simulink model "integration_2-1"  (R2023b)
settings: Solver=FixedStepAuto  StartTime=0.0  StopTime=inf  FixedStep=0.01  RelTol=1e-3  EnableMultiTasking=on
InitFcn:
  | params
  | pin_params
undefined symbols (not defined in the file): b, default1, den_Gd, encoder_scale, f, J, Kb, KD, Kf, KI, Km, KP, l, L, num_Gd, r, R, steering, Vlim
libraries: arduinolib x18, arduinosensorlib x8, simulink x2
settings Model: SimulationMode=external  ExtModeTrigDuration=2  Creator=권주성  LastModifiedBy=tkdle
settings SolverCC: AutoInsertRateTranBlk=on
settings OptimizationCC: EnhancedBackFolding=on  PassReuseOutputArgsAs=Individual arguments  ZeroExternalMemoryAtStartup=off  ZeroInternalMemoryAtStartup=off  MaxStackSize=64  OptimizeBlockOrder=speed  DifferentSizesBufferReuse=on  OptimizationCustomize=off  EfficientTunableParamExpr=on
settings DebuggingCC: ParameterPrecisionLossMsg=none  ParameterTunabilityLossMsg=error
settings HardwareCC: ProdBitPerInt=16  ProdBitPerPointer=16  ProdBitPerSizeT=16  ProdBitPerPtrDiffT=16  ProdLargestAtomicFloat=None  ProdWordSize=8  ProdHWDeviceType=Atmel->AVR
settings SFSimCC: MATLABDynamicMemAlloc=off
settings RTWCC: Description=Embedded Coder  SystemTargetFile=ert.tlc  HardwareBoard=Arduino Mega 2560  TemplateMakefile=ert_default_tmf  Toolchain=Arduino AVR  BuildConfiguration=Faster Runs
settings CodeAppCC: ForceParamTrailComments=on  IgnoreCustomStorageClasses=off  OperatorAnnotations=on  SimulinkDataObjDesc=on  SFDataObjDesc=on  InsertBlockDesc=on
settings ERTTargetCC: SupportContinuousTime=on  SupportVariableSizeSignals=on  ExtMode=on  ExtModeTransport=3  ExtModeStaticAlloc=on  ExtModeAutomaticAllocSize=off  ExtModeStaticAllocSize=2048  ExtModeMexFile=ext_xcp  ExtModeMexArgs=0 12 921600  ExtModeIntrfLevel=Level2 - Open

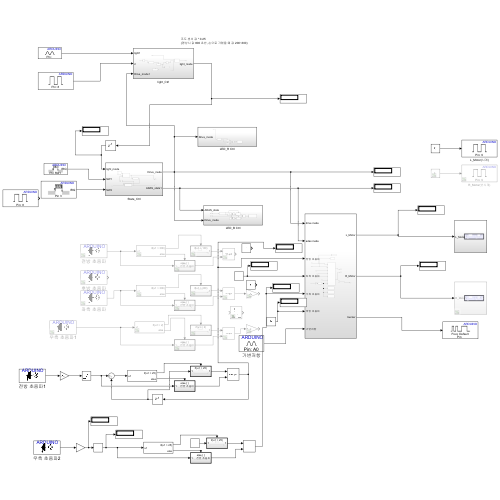
[thumbnail: Simulink's stored preview of the top-level diagram]
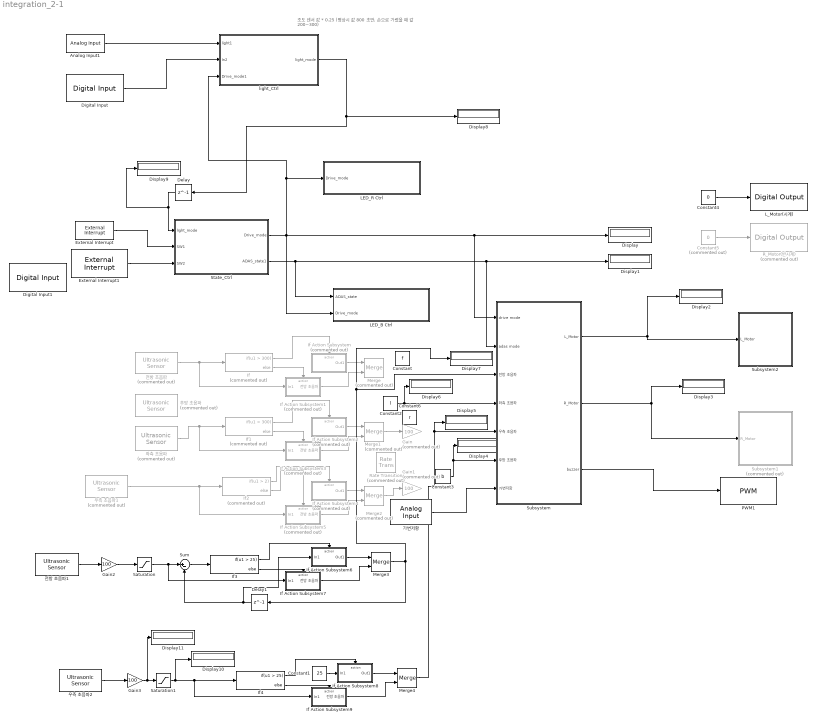
== system integration_2-1 ==
  note: 조도 센서 값 * 0.25
      | (평상시 값 800 초반, 손으로 가렸을 때 값 200~300)
  Analog Input1 : arduinolib/Analog Input  pinNumber=BS  ReadResultsOnly=off  ConversionTriggerSource=Software  ExternalTriggerType=uint32( 0 )  OutputDataType=uint16  EnableConversionCompleteNotify=off  EnableOuputStatus=off  SampleTime=-1  blockPlatform=arduino
  Constant : Constant  Value=f
  Constant1 : Constant  Value=25
  Constant2 : Constant  Value=l
  Constant3 : Constant  Value=b
  Constant4 : Constant  Value=0
  Constant5 : Constant  Commented=on  Value=0
  Constant6 : Constant  Value=r
  Delay : Delay  DelayLength=1
  Delay1 : Delay  DelayLength=1
  Digital Input : arduinolib/Digital Input  pinNumber=SW3  mode=Default  Direction=input  SampleTime=0.1  blockPlatform=arduino
  Digital Input1 : arduinolib/Digital Input  pinNumber=SW2  mode=Default  Direction=input  SampleTime=0.1  blockPlatform=arduino
  Display{,1..11} (12 alike) : Display
  External Interrupt : arduinolib/External Interrupt  Pin=SW1  PullUp=off  Mode=RISING  InterruptSimulationInput=off
  External Interrupt1 : arduinolib/External Interrupt  Pin=3  PullUp=off  Mode=RISING  InterruptSimulationInput=off
  Gain : Gain  Commented=on  Gain=100
  Gain1 : Gain  Commented=on  Gain=100
  Gain2 : Gain  Gain=100
  Gain3 : Gain  Gain=100
  If : If  Commented=on  IfExpression=u1 > 300
  If Action Subsystem : Subsystem  Commented=on  TreatAsAtomicUnit=on
  If Action Subsystem1 : Subsystem  Commented=on  TreatAsAtomicUnit=on
  If Action Subsystem2 : Subsystem  Commented=on  TreatAsAtomicUnit=on
  If Action Subsystem3 : Subsystem  Commented=on  TreatAsAtomicUnit=on
  If Action Subsystem4 : Subsystem  Commented=on  TreatAsAtomicUnit=on
  If Action Subsystem5 : Subsystem  Commented=on  TreatAsAtomicUnit=on
  If Action Subsystem6 : Subsystem  TreatAsAtomicUnit=on
  If Action Subsystem7 : Subsystem  TreatAsAtomicUnit=on
  If Action Subsystem8 : Subsystem  TreatAsAtomicUnit=on
  If Action Subsystem9 : Subsystem  TreatAsAtomicUnit=on
  If1 : If  Commented=on  IfExpression=u1 > 300
  If2 : If  Commented=on  IfExpression=u1 > 2
  If3 : If  IfExpression=u1 > 25
  If4 : If  IfExpression=u1 > 25
  LED_B Ctrl : Subsystem
  LED_R Ctrl : Subsystem
  L_Motor(시계) : arduinolib/Digital Output  pinNumber=Motor_L_Direction  Direction=output  blockPlatform=arduino
  Merge : Merge  Commented=on
  Merge1 : Merge  Commented=on
  Merge2 : Merge  Commented=on
  Merge3 : Merge
  Merge4 : Merge
  PWM1 : arduinolib/PWM  pinNumber=Buzzer  frequencyType=Default  desiredFrequency=490.2  achievableFrequency=490.2
  R_Motor(반시계) : arduinolib/Digital Output  Commented=on  pinNumber=Motor_R_Direction  Direction=output  blockPlatform=arduino
  Rate Transition : RateTransition  Commented=on  Integrity=off  OutPortSampleTime=0.01
  Saturation : Saturate  UpperLimit=30  LowerLimit=0
  Saturation1 : Saturate  UpperLimit=30
  State_Ctrl : Subsystem
  Subsystem : Subsystem
  Subsystem1 : Subsystem  Commented=on
  Subsystem2 : Subsystem
  Sum : Sum  Inputs=|+-
  light_Ctrl : Subsystem
  가변저항 : arduinolib/Analog Input  pinNumber=0  ReadResultsOnly=off  ConversionTriggerSource=Software  ExternalTriggerType=uint32( 0 )  OutputDataType=uint16  EnableConversionCompleteNotify=off  EnableOuputStatus=off  SampleTime=-1  blockPlatform=arduino
  우측 초음파1 : arduinosensorlib/Ultrasonic Sensor  Commented=on  NumSignalPins=2  TrigPin=R_Triger  EchoPin=R_Echo  SignalPin=3  SampleTime_=0.01  blockPlatform=ARDUINO
  우측 초음파2 : arduinosensorlib/Ultrasonic Sensor  NumSignalPins=2  TrigPin=R_Triger  EchoPin=R_Echo  SignalPin=3  SampleTime_=0.01  blockPlatform=ARDUINO
  전방 초음파 : arduinosensorlib/Ultrasonic Sensor  Commented=on  NumSignalPins=2  TrigPin=F_Triger  EchoPin=F_Echo  SignalPin=3  SampleTime_=0.01  blockPlatform=ARDUINO
  전방 초음파1 : arduinosensorlib/Ultrasonic Sensor  NumSignalPins=2  TrigPin=F_Triger  EchoPin=F_Echo  SignalPin=3  SampleTime_=0.01  blockPlatform=ARDUINO
  좌측 초음파 : arduinosensorlib/Ultrasonic Sensor  Commented=on  NumSignalPins=2  TrigPin=L_Triger  EchoPin=L_Echo  SignalPin=3  SampleTime_=0.01  blockPlatform=ARDUINO
  후방 초음파 : arduinosensorlib/Ultrasonic Sensor  Commented=on  NumSignalPins=2  TrigPin=B_Triger  EchoPin=B_Echo  SignalPin=3  SampleTime_=0.01  blockPlatform=ARDUINO
  wires:
  light_Ctrl/1(light_mode) -> Display8/1, Delay/1
  Analog Input1/1 -> light_Ctrl/1(light1)
  Delay/1 -> Display9/1, State_Ctrl/1(light_mode)
  State_Ctrl/2(ADAS_state1) -> LED_B Ctrl/1(ADAS_state), Display1/1, Subsystem/2(adas mode)
  External Interrupt/1 -> State_Ctrl/2(SW1)
  State_Ctrl/1(Drive_mode) -> Subsystem/1(drive mode), Display/1, light_Ctrl/3(Drive_mode1), LED_R Ctrl/1(Drive_mode), LED_B Ctrl/2(Drive_mode)
  가변저항/1 -> Subsystem/7(가변저항)
  Subsystem/3(buzzer) -> PWM1/1
  Subsystem/2(R_Motor) -> Subsystem1/1(R_Motor), Display3/1
  Merge1/1 -> Gain/1
  Constant2/1 -> Subsystem/4(좌측 초음파), Display6/1
  Subsystem/1(L_Motor) -> Display2/1, Subsystem2/1(L_Motor)
  External Interrupt1/1 -> State_Ctrl/3(SW2)
  Digital Input/1 -> light_Ctrl/2(In2)
  Constant4/1 -> L_Motor(시계)/1
  Constant5/1 -> R_Motor(반시계)/1
  전방 초음파/1 -> If Action Subsystem1/1(In1), If/1
  If/1 -> If Action Subsystem/Action
  If/2 -> If Action Subsystem1/Action
  If Action Subsystem/1(Out1) -> Merge/1
  If Action Subsystem1/1(전방 초음파) -> Merge/2
  좌측 초음파/1 -> If Action Subsystem3/1(In1), If1/1
  If1/1 -> If Action Subsystem2/Action
  If1/2 -> If Action Subsystem3/Action
  If Action Subsystem2/1(Out1) -> Merge1/1
  If Action Subsystem3/1(전방 초음파) -> Merge1/2
  If Action Subsystem5/1(전방 초음파) -> Merge2/2
  If Action Subsystem4/1(Out1) -> Merge2/1
  If2/2 -> If Action Subsystem5/Action
  If2/1 -> If Action Subsystem4/Action
  Merge2/1 -> Gain1/1
  우측 초음파1/1 -> If Action Subsystem5/1(In1), If2/1
  전방 초음파1/1 -> Gain2/1
  Gain2/1 -> Saturation/1
  Saturation/1 -> If Action Subsystem7/1(In1), Sum/1
  Merge3/1 -> Subsystem/3(전방 초음파), Display7/1, Delay1/1
  Delay1/1 -> If Action Subsystem6/1(In1), Sum/2
  Sum/1 -> If3/1
  If3/1 -> If Action Subsystem6/Action
  If3/2 -> If Action Subsystem7/Action
  If Action Subsystem6/1(Out1) -> Merge3/1
  If Action Subsystem7/1(전방 초음파) -> Merge3/2
  Constant3/1 -> Display4/1, Subsystem/6(후방 초음파)
  우측 초음파2/1 -> Gain3/1
  If Action Subsystem8/1(Out1) -> Merge4/1
  If4/1 -> If Action Subsystem8/Action
  If Action Subsystem9/1(전방 초음파) -> Merge4/2
  Saturation1/1 -> Display10/1, If4/1, If Action Subsystem9/1(In1)
  Gain3/1 -> Display11/1, Saturation1/1
  Merge4/1 -> Display5/1, Subsystem/5(우측 초음파)
  If4/2 -> If Action Subsystem9/Action
  Constant1/1 -> If Action Subsystem8/1(In1)

== system integration_2-1/If Action Subsystem ==
  Action Port : ActionPort  ActionPortLabel=if(u1 > 100)
  Constant : Constant  Value=f
  Out1 : Outport
  wires:
  Constant/1 -> Out1/1

== system integration_2-1/If Action Subsystem1 ==
  In1 : Inport
  Action Port : ActionPort  ActionPortLabel=else
  전방 초음파 : Outport
  wires:
  In1/1 -> 전방 초음파/1

== system integration_2-1/If Action Subsystem2 ==
  Action Port : ActionPort  ActionPortLabel=if(u1 > 300)
  Constant : Constant  Value=300
  Out1 : Outport
  wires:
  Constant/1 -> Out1/1

== system integration_2-1/If Action Subsystem3 ==
  In1 : Inport
  Action Port : ActionPort  ActionPortLabel=else
  전방 초음파 : Outport
  wires:
  In1/1 -> 전방 초음파/1

== system integration_2-1/If Action Subsystem4 ==
  Action Port : ActionPort  ActionPortLabel=if(u1 > 2)
  Constant : Constant  Value=2
  Out1 : Outport
  wires:
  Constant/1 -> Out1/1

== system integration_2-1/If Action Subsystem5 ==
  In1 : Inport
  Action Port : ActionPort  ActionPortLabel=else
  전방 초음파 : Outport
  wires:
  In1/1 -> 전방 초음파/1

== system integration_2-1/If Action Subsystem6 ==
  In1 : Inport
  Action Port : ActionPort  ActionPortLabel=if(u1 > 25)
  Out1 : Outport
  wires:
  In1/1 -> Out1/1

== system integration_2-1/If Action Subsystem7 ==
  In1 : Inport
  Action Port : ActionPort  ActionPortLabel=else
  전방 초음파 : Outport
  wires:
  In1/1 -> 전방 초음파/1

== system integration_2-1/If Action Subsystem8 ==
  In1 : Inport
  Action Port : ActionPort  ActionPortLabel=if(u1 > 25)
  Out1 : Outport
  wires:
  In1/1 -> Out1/1

== system integration_2-1/If Action Subsystem9 ==
  In1 : Inport
  Action Port : ActionPort  ActionPortLabel=else
  전방 초음파 : Outport
  wires:
  In1/1 -> 전방 초음파/1

== system integration_2-1/LED_B Ctrl ==
  ADAS_state : Inport
  Drive_mode : Inport  Port=2
  Constant : Constant
  Digital Output : arduinolib/Digital Output  pinNumber=LED1_B  Direction=output  blockPlatform=arduino
  If Action Subsystem1 : Subsystem  TreatAsAtomicUnit=on
  If Action Subsystem3 : Subsystem  TreatAsAtomicUnit=on
  If1 : If  IfExpression=u1 ==1
  Merge : Merge
  Product : Product
  Product1 : Product
  Pulse Generator : DiscretePulseGenerator  PulseType=Time based  PulseWidth=50
  wires:
  If1/2 -> If Action Subsystem3/Action
  If Action Subsystem1/1(Out1) -> Merge/1
  ADAS_state/1 -> If1/1
  If1/1 -> If Action Subsystem1/Action
  Merge/1 -> Digital Output/1
  If Action Subsystem3/1(Out1) -> Merge/2
  Drive_mode/1 -> Product/1, Product1/2
  Pulse Generator/1 -> Product/2
  Constant/1 -> Product1/1
  Product1/1 -> If Action Subsystem1/1(Input)
  Product/1 -> If Action Subsystem3/1(Input)

== system integration_2-1/LED_R Ctrl ==
  Drive_mode : Inport
  Digital Output : arduinolib/Digital Output  pinNumber=LED1_R  Direction=output  blockPlatform=arduino
  If Action Subsystem1 : Subsystem  TreatAsAtomicUnit=on
  If Action Subsystem3 : Subsystem  TreatAsAtomicUnit=on
  If1 : If  IfExpression=u1 ==1
  Merge : Merge
  wires:
  If1/2 -> If Action Subsystem3/Action
  If Action Subsystem1/1(Out1) -> Merge/1
  Drive_mode/1 -> If1/1
  If1/1 -> If Action Subsystem1/Action
  Merge/1 -> Digital Output/1
  If Action Subsystem3/1(Out1) -> Merge/2

== system integration_2-1/State_Ctrl ==
  light_mode : Inport
  SW1 : Inport  Port=2
  SW2 : Inport  Port=3
  ADAS_state : Subsystem
  Delay : Delay  DelayLength=1
  If : If  IfExpression=u1 ==1  ShowElse=off
  drive_mode : Subsystem
  Drive_mode : Outport
  ADAS_state1 : Outport  Port=2
  wires:
  If/1 -> ADAS_state/1(In1)
  drive_mode/1(D_mode) -> If/1, Drive_mode/1
  ADAS_state/1(ADAS_state) -> Delay/1, ADAS_state1/1
  SW1/1 -> drive_mode/2(sw1)
  Delay/1 -> drive_mode/3(A_state)
  light_mode/1 -> drive_mode/1(light_mode)
  SW2/1 -> ADAS_state/2(In2)

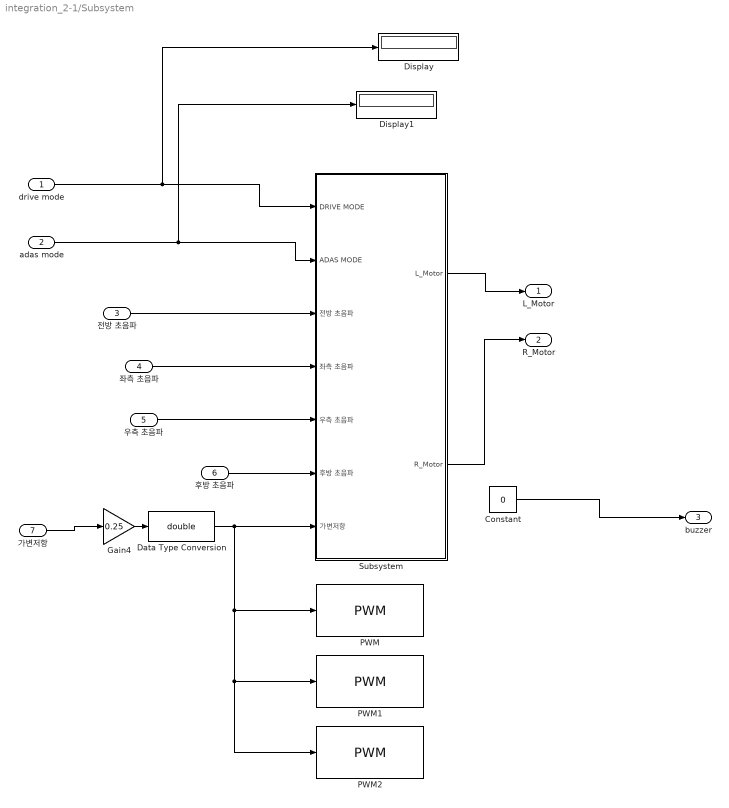
== system integration_2-1/Subsystem ==
  drive mode : Inport
  adas mode : Inport  Port=2
  전방 초음파 : Inport  Port=3
  좌측 초음파 : Inport  Port=4
  우측 초음파 : Inport  Port=5
  후방 초음파 : Inport  Port=6
  가변저항 : Inport  Port=7
  Constant : Constant  Value=0
  Data Type Conversion : DataTypeConversion  OutDataTypeStr=double  SaturateOnIntegerOverflow=off  RndMeth=Floor
  Display : Display
  Display1 : Display
  Gain4 : Gain  Gain=0.25
  PWM : arduinolib/PWM  pinNumber=RGB_LED_1  frequencyType=Default  desiredFrequency=490.2  achievableFrequency=490.2
  PWM1 : arduinolib/PWM  pinNumber=RGB_LED_2  frequencyType=Default  desiredFrequency=490.2  achievableFrequency=490.2
  PWM2 : arduinolib/PWM  pinNumber=RGB_LED_3  frequencyType=Default  desiredFrequency=490.2  achievableFrequency=490.2
  Subsystem : Subsystem
  L_Motor : Outport
  R_Motor : Outport  Port=2
  buzzer : Outport  Port=3
  wires:
  drive mode/1 -> Subsystem/1(DRIVE MODE), Display/1
  adas mode/1 -> Subsystem/2(ADAS MODE), Display1/1
  Constant/1 -> buzzer/1
  가변저항/1 -> Gain4/1
  Gain4/1 -> Data Type Conversion/1
  Data Type Conversion/1 -> Subsystem/7(가변저항), PWM2/1, PWM1/1, PWM/1
  Subsystem/1(L_Motor) -> L_Motor/1
  Subsystem/2(R_Motor) -> R_Motor/1
  전방 초음파/1 -> Subsystem/3(전방 초음파)
  좌측 초음파/1 -> Subsystem/4(좌측 초음파)
  우측 초음파/1 -> Subsystem/5(우측 초음파)
  후방 초음파/1 -> Subsystem/6(후방 초음파)

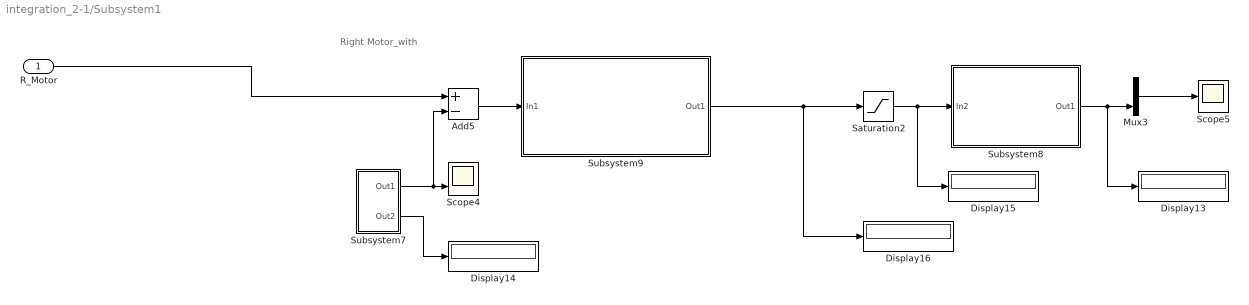
== system integration_2-1/Subsystem1 ==
  note: Right Motor_with
  R_Motor : Inport
  Add5 : Sum  Inputs=+-
  Display{13..16} (4 alike) : Display
  Mux3 : Mux  Inputs=2
  Saturation2 : Saturate  UpperLimit=12  LowerLimit=0
  Scope4 : Scope  NumInputPorts=2
  Scope5 : Scope
  Subsystem7 : Subsystem
  Subsystem8 : Subsystem
  Subsystem9 : Subsystem
  wires:
  Mux3/1 -> Scope5/1
  Saturation2/1 -> Subsystem8/1(In2), Display15/1
  Subsystem9/1(Out1) -> Display16/1, Saturation2/1
  Subsystem8/1(Out1) -> Display13/1, Mux3/2
  Subsystem7/1(Out1) -> Add5/2, Scope4/2
  Subsystem7/2(Out2) -> Display14/1
  Add5/1 -> Subsystem9/1(In1)
  R_Motor/1 -> Add5/1

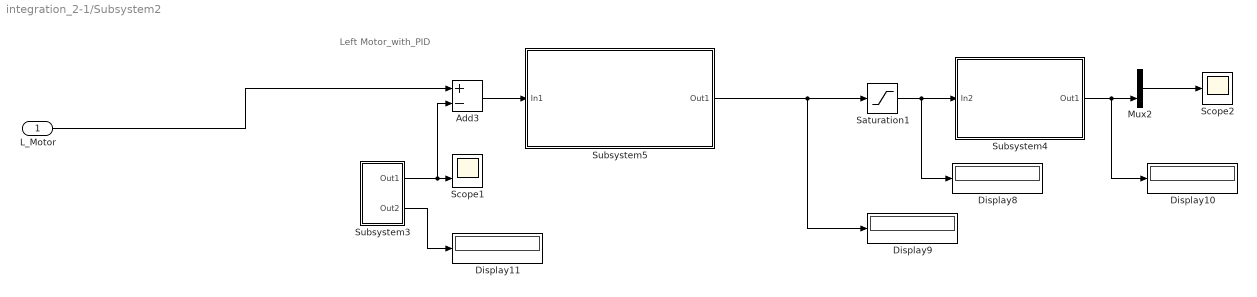
== system integration_2-1/Subsystem2 ==
  note: Left Motor_with_PID
  L_Motor : Inport
  Add3 : Sum  Inputs=+-
  Display{8..11} (4 alike) : Display
  Mux2 : Mux  Inputs=2
  Saturation1 : Saturate  UpperLimit=12  LowerLimit=0
  Scope1 : Scope  NumInputPorts=2
  Scope2 : Scope
  Subsystem3 : Subsystem
  Subsystem4 : Subsystem
  Subsystem5 : Subsystem
  wires:
  Mux2/1 -> Scope2/1
  Saturation1/1 -> Subsystem4/1(In2), Display8/1
  Subsystem5/1(Out1) -> Display9/1, Saturation1/1
  Subsystem3/2(Out2) -> Display11/1
  Add3/1 -> Subsystem5/1(In1)
  Subsystem3/1(Out1) -> Add3/2, Scope1/2
  Subsystem4/1(Out1) -> Display10/1, Mux2/2
  L_Motor/1 -> Add3/1

== system integration_2-1/light_Ctrl ==
  light1 : Inport
  In2 : Inport  Port=2
  Drive_mode1 : Inport  Port=3
  Display1 : Display
  Function-Call Subsystem1 : Subsystem  Commented=on  TreatAsAtomicUnit=on
  If : If  IfExpression=u1 == 0  ShowElse=off
  If Action Subsystem : Subsystem  TreatAsAtomicUnit=on
  Rate Transition : RateTransition  Integrity=off
  Rate Transition1 : RateTransition  Integrity=off  OutPortSampleTime=0.2
  Subsystem : Subsystem
  light_mode : Outport
  wires:
  If Action Subsystem/1(Out1) -> Display1/1, Rate Transition/1
  In2/1 -> Rate Transition1/1
  Rate Transition/1 -> Subsystem/2(sw3)
  Drive_mode1/1 -> Subsystem/3(Drive_mode1)
  light1/1 -> Subsystem/1(light1)
  Subsystem/1(light_mode) -> light_mode/1
  If/1 -> If Action Subsystem/Action
  Rate Transition1/1 -> If/1

== system integration_2-1/LED_B Ctrl/If Action Subsystem1 ==
  Input : Inport
  Action Port : ActionPort  ActionPortLabel=if(u1 ==1)
  Out1 : Outport
  wires:
  Input/1 -> Out1/1

== system integration_2-1/LED_B Ctrl/If Action Subsystem3 ==
  Input : Inport
  Action Port : ActionPort  ActionPortLabel=else
  Out1 : Outport
  wires:
  Input/1 -> Out1/1

== system integration_2-1/LED_R Ctrl/If Action Subsystem1 ==
  Action Port : ActionPort  ActionPortLabel=if(u1 ==1)
  Constant : Constant
  Out1 : Outport
  wires:
  Constant/1 -> Out1/1

== system integration_2-1/LED_R Ctrl/If Action Subsystem3 ==
  Action Port : ActionPort  ActionPortLabel=else
  Constant : Constant  Value=0
  Out1 : Outport
  wires:
  Constant/1 -> Out1/1

== system integration_2-1/State_Ctrl/ADAS_state ==
  In1 : Inport
  In2 : Inport  Port=2
  If Action Subsystem : Subsystem  TreatAsAtomicUnit=on
  Rate Transition2 : RateTransition  Integrity=off
  SW2 : Subsystem
  ADAS_state : Outport
  wires:
  In1/1 -> If Action Subsystem/Action
  If Action Subsystem/1(ADAS_state) -> ADAS_state/1
  In2/1 -> SW2/Trigger
  SW2/1(SW2) -> Rate Transition2/1
  Rate Transition2/1 -> If Action Subsystem/1(sw2)

== system integration_2-1/State_Ctrl/drive_mode ==
  light_mode : Inport
  sw1 : Inport  Port=2
  A_state : Inport  Port=3
  Chart : Stateflow chart  TreatAsAtomicUnit=on
  Rate Transition : RateTransition  Integrity=off
  SW1 : Subsystem
  D_mode : Outport
  wires:
  SW1/1(Output) -> Rate Transition/1
  Rate Transition/1 -> Chart/1(sw1)
  Chart/1(drive_mode) -> D_mode/1
  sw1/1 -> SW1/Trigger
  A_state/1 -> Chart/3(A_state)
  light_mode/1 -> Chart/2(light_mode)

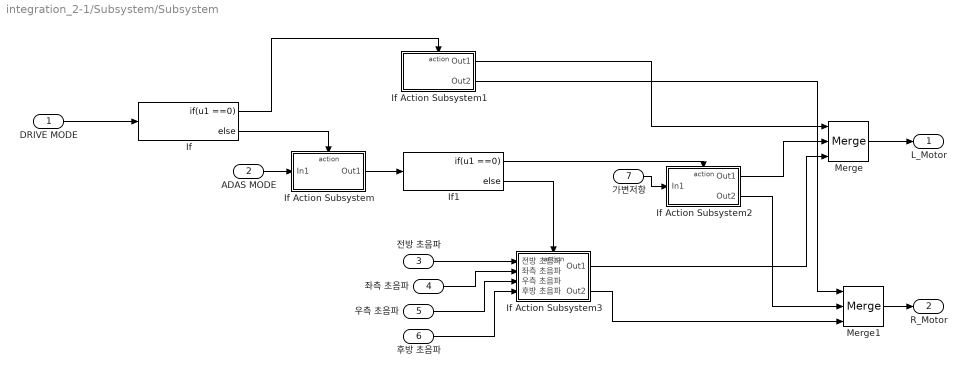
== system integration_2-1/Subsystem/Subsystem ==
  DRIVE MODE : Inport
  ADAS MODE : Inport  Port=2
  전방 초음파 : Inport  Port=3
  좌측 초음파 : Inport  Port=4
  우측 초음파 : Inport  Port=5
  후방 초음파 : Inport  Port=6
  가변저항 : Inport  Port=7
  If : If  IfExpression=u1 ==0
  If Action Subsystem : Subsystem  TreatAsAtomicUnit=on
  If Action Subsystem1 : Subsystem  TreatAsAtomicUnit=on
  If Action Subsystem2 : Subsystem  TreatAsAtomicUnit=on
  If Action Subsystem3 : Subsystem  TreatAsAtomicUnit=on
  If1 : If  IfExpression=u1 ==0
  Merge : Merge  Inputs=3
  Merge1 : Merge  Inputs=3
  L_Motor : Outport
  R_Motor : Outport  Port=2
  wires:
  DRIVE MODE/1 -> If/1
  If/2 -> If Action Subsystem/Action
  If/1 -> If Action Subsystem1/Action
  ADAS MODE/1 -> If Action Subsystem/1(In1)
  If Action Subsystem/1(Out1) -> If1/1
  If1/1 -> If Action Subsystem2/Action
  가변저항/1 -> If Action Subsystem2/1(In1)
  If1/2 -> If Action Subsystem3/Action
  If Action Subsystem1/1(Out1) -> Merge/1
  If Action Subsystem2/1(Out1) -> Merge/2
  If Action Subsystem3/1(Out1) -> Merge/3
  If Action Subsystem1/2(Out2) -> Merge1/1
  If Action Subsystem2/2(Out2) -> Merge1/2
  If Action Subsystem3/2(Out2) -> Merge1/3
  Merge/1 -> L_Motor/1
  Merge1/1 -> R_Motor/1
  전방 초음파/1 -> If Action Subsystem3/1(전방 초음파)
  좌측 초음파/1 -> If Action Subsystem3/2(좌측 초음파)
  우측 초음파/1 -> If Action Subsystem3/3(우측 초음파)
  후방 초음파/1 -> If Action Subsystem3/4(후방 초음파)

== system integration_2-1/Subsystem1/Subsystem7 ==
  Data Type Conversion1 : DataTypeConversion  OutDataTypeStr=int32  SaturateOnIntegerOverflow=off  RndMeth=Floor
  Discrete Transfer Fcn : DiscreteTransferFcn  Numerator=num_Gd  Denominator=den_Gd
  Discrete Derivative : simulink/Discrete/Discrete Derivative  gainval=1.0  ICPrevScaledInput=0.0  OutMin=[]  OutMax=[]  OutDataType=fixdt(1, 16)  OutScaling=2^-10  DoSatur=off
  Display : Display
  Encoder : arduinosensorlib/Encoder  InputA=R_Encoder_A  InputB=R_Encoder_B  Mode=No reset  SampleTime=-1
  Gain1 : Gain  Gain=encoder_scale
  Gain2 : Gain  Gain=60/(2*pi)
  Out1 : Outport
  Out2 : Outport  Port=2
  wires:
  Gain1/1 -> Display/1, Gain2/1, Data Type Conversion1/1
  Encoder/1 -> Discrete Derivative/1
  Gain2/1 -> Out2/1
  Data Type Conversion1/1 -> Discrete Transfer Fcn/1
  Discrete Derivative/1 -> Gain1/1
  Discrete Transfer Fcn/1 -> Out1/1

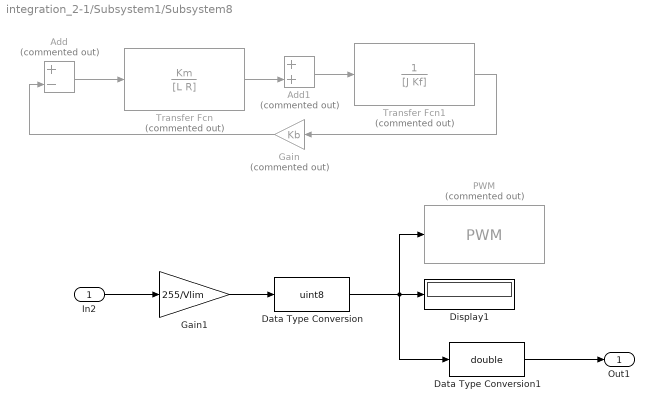
== system integration_2-1/Subsystem1/Subsystem8 ==
  In2 : Inport
  Add : Sum  Commented=on  Inputs=+-
  Add1 : Sum  Commented=on
  Data Type Conversion : DataTypeConversion  OutDataTypeStr=uint8  SaturateOnIntegerOverflow=off  RndMeth=Floor
  Data Type Conversion1 : DataTypeConversion  OutDataTypeStr=double  SaturateOnIntegerOverflow=off  RndMeth=Floor
  Display1 : Display
  Gain : Gain  Commented=on  Gain=Kb
  Gain1 : Gain  Gain=255/Vlim
  PWM : arduinolib/PWM  Commented=on  pinNumber=Motor_R_control  frequencyType=Default  desiredFrequency=490.2  achievableFrequency=490.2
  Transfer Fcn : TransferFcn  Commented=on  Numerator=Km  Denominator=[L R]
  Transfer Fcn1 : TransferFcn  Commented=on  Numerator=1  Denominator=[J Kf]
  Out1 : Outport
  wires:
  ? -> Add/1
  ? -> Add1/1
  Add/1 -> Transfer Fcn/1
  Add1/1 -> Transfer Fcn1/1
  Transfer Fcn/1 -> Add1/2
  Gain/1 -> Add/2
  Transfer Fcn1/1 -> Gain/1
  In2/1 -> Gain1/1
  Gain1/1 -> Data Type Conversion/1
  Data Type Conversion1/1 -> Out1/1
  Data Type Conversion/1 -> Data Type Conversion1/1, Display1/1, PWM/1

== system integration_2-1/Subsystem1/Subsystem9 ==
  In1 : Inport
  Derivative2 : Derivative
  Gain1 : Gain  Gain=KI
  Gain2 : Gain  Gain=KP
  Gain3 : Gain  Gain=KD
  Integrator2 : Integrator
  Subtract2 : Sum  Inputs=+++
  Out1 : Outport
  wires:
  Gain1/1 -> Integrator2/1
  Gain2/1 -> Subtract2/2
  Integrator2/1 -> Subtract2/1
  In1/1 -> Gain2/1, Gain3/1, Gain1/1
  Derivative2/1 -> Subtract2/3
  Gain3/1 -> Derivative2/1
  Subtract2/1 -> Out1/1

== system integration_2-1/Subsystem2/Subsystem3 ==
  Data Type Conversion1 : DataTypeConversion  OutDataTypeStr=int32  SaturateOnIntegerOverflow=off  RndMeth=Floor
  Discrete Transfer Fcn : DiscreteTransferFcn  Numerator=num_Gd  Denominator=den_Gd
  Discrete Derivative : simulink/Discrete/Discrete Derivative  gainval=1.0  ICPrevScaledInput=0.0  OutMin=[]  OutMax=[]  OutDataType=fixdt(1, 16)  OutScaling=2^-10  DoSatur=off
  Display : Display
  Encoder : arduinosensorlib/Encoder  InputA=L_Encoder_A  InputB=L_Encoder_B  Mode=No reset  SampleTime=-1
  Gain1 : Gain  Gain=encoder_scale
  Gain2 : Gain  Gain=60/(2*pi)
  Out1 : Outport
  Out2 : Outport  Port=2
  wires:
  Gain1/1 -> Display/1, Gain2/1, Data Type Conversion1/1
  Encoder/1 -> Discrete Derivative/1
  Gain2/1 -> Out2/1
  Data Type Conversion1/1 -> Discrete Transfer Fcn/1
  Discrete Derivative/1 -> Gain1/1
  Discrete Transfer Fcn/1 -> Out1/1

== system integration_2-1/Subsystem2/Subsystem4 ==
  In2 : Inport
  Add : Sum  Commented=on  Inputs=+-
  Add1 : Sum  Commented=on
  Data Type Conversion : DataTypeConversion  OutDataTypeStr=uint8  SaturateOnIntegerOverflow=off  RndMeth=Floor
  Data Type Conversion1 : DataTypeConversion  OutDataTypeStr=double  SaturateOnIntegerOverflow=off  RndMeth=Floor
  Display1 : Display
  Gain : Gain  Commented=on  Gain=Kb
  Gain1 : Gain  Gain=255/Vlim
  PWM : arduinolib/PWM  pinNumber=Motor_L_Control  frequencyType=Default  desiredFrequency=490.2  achievableFrequency=490.2
  Transfer Fcn : TransferFcn  Commented=on  Numerator=Km  Denominator=[L R]
  Transfer Fcn1 : TransferFcn  Commented=on  Numerator=1  Denominator=[J Kf]
  Out1 : Outport
  wires:
  ? -> Add/1
  ? -> Add1/1
  Add/1 -> Transfer Fcn/1
  Add1/1 -> Transfer Fcn1/1
  Transfer Fcn/1 -> Add1/2
  Gain/1 -> Add/2
  Transfer Fcn1/1 -> Gain/1
  In2/1 -> Gain1/1
  Gain1/1 -> Data Type Conversion/1
  Data Type Conversion1/1 -> Out1/1
  Data Type Conversion/1 -> Data Type Conversion1/1, Display1/1, PWM/1

== system integration_2-1/Subsystem2/Subsystem5 ==
  In1 : Inport
  Derivative2 : Derivative
  Gain1 : Gain  Gain=KI
  Gain2 : Gain  Gain=KP
  Gain3 : Gain  Gain=KD
  Integrator2 : Integrator
  Subtract2 : Sum  Inputs=+++
  Out1 : Outport
  wires:
  Gain1/1 -> Integrator2/1
  Gain2/1 -> Subtract2/2
  Integrator2/1 -> Subtract2/1
  In1/1 -> Gain2/1, Gain3/1, Gain1/1
  Derivative2/1 -> Subtract2/3
  Gain3/1 -> Derivative2/1
  Subtract2/1 -> Out1/1

== system integration_2-1/light_Ctrl/Function-Call Subsystem1 ==
  function : TriggerPort  TriggerType=function-call  VariantControl=(inherit)
  Constant : Constant
  Constant1 : Constant  Value=3
  Delay : Delay  DelayLength=1
  Mod : Math  Operator=mod
  Sum : Sum  Inputs=|++
  Output : Outport
  wires:
  Constant/1 -> Sum/1
  Delay/1 -> Sum/2
  Constant1/1 -> Mod/2
  Sum/1 -> Delay/1, Mod/1
  Mod/1 -> Output/1

== system integration_2-1/light_Ctrl/If Action Subsystem ==
  Action Port : ActionPort  ActionPortLabel=if(u1 == 0)
  Constant : Constant
  Constant1 : Constant  Value=3
  Delay : Delay  DelayLength=1
  Mod : Math  Operator=mod
  Plus : Sum
  Out1 : Outport
  wires:
  Mod/1 -> Out1/1, Delay/1
  Constant/1 -> Plus/1
  Delay/1 -> Plus/2
  Plus/1 -> Mod/1
  Constant1/1 -> Mod/2

== system integration_2-1/light_Ctrl/Subsystem ==
  light1 : Inport
  sw3 : Inport  Port=2
  Drive_mode1 : Inport  Port=3
  Chart1 : Stateflow chart  TreatAsAtomicUnit=on
  Subsystem : Subsystem
  light_mode : Outport
  wires:
  Chart1/1(light_mode) -> Subsystem/2(light_mode), light_mode/1
  light1/1 -> Subsystem/1(light)
  sw3/1 -> Chart1/1(sw3)
  Drive_mode1/1 -> Chart1/2(Drive_mode)

== system integration_2-1/State_Ctrl/ADAS_state/If Action Subsystem ==
  sw2 : Inport
  Action Port : ActionPort  ActionPortLabel=if(u1 ==1)
  Chart : Stateflow chart  TreatAsAtomicUnit=on
  ADAS_state : Outport
  wires:
  sw2/1 -> Chart/1(sw2)
  Chart/1(ADAS_state) -> ADAS_state/1

== system integration_2-1/State_Ctrl/ADAS_state/SW2 ==
  function : TriggerPort  TriggerType=function-call  VariantControl=(inherit)
  Constant : Constant
  Constant1 : Constant  Value=2
  Delay : Delay  DelayLength=1  InitialCondition=0
  Mod : Math  Operator=mod
  Sum : Sum  Inputs=|++
  SW2 : Outport
  wires:
  Sum/1 -> Delay/1, Mod/1
  Constant1/1 -> Mod/2
  Mod/1 -> SW2/1
  Constant/1 -> Sum/1
  Delay/1 -> Sum/2

== system integration_2-1/State_Ctrl/drive_mode/SW1 ==
  function : TriggerPort  TriggerType=function-call  VariantControl=(inherit)
  Constant : Constant
  Constant1 : Constant  Value=2
  Delay : Delay  DelayLength=1
  Mod : Math  Operator=mod
  Sum : Sum  Inputs=|++
  Output : Outport
  wires:
  Constant/1 -> Sum/1
  Sum/1 -> Delay/1, Mod/1
  Constant1/1 -> Mod/2
  Delay/1 -> Sum/2
  Mod/1 -> Output/1

== system integration_2-1/Subsystem/Subsystem/If Action Subsystem ==
  In1 : Inport
  Action Port : ActionPort  ActionPortLabel=else
  Out1 : Outport
  wires:
  In1/1 -> Out1/1

== system integration_2-1/Subsystem/Subsystem/If Action Subsystem1 ==
  Action Port : ActionPort  ActionPortLabel=if(u1 ==0)
  Constant : Constant  Value=0
  Constant1 : Constant  Value=0
  Out1 : Outport
  Out2 : Outport  Port=2
  wires:
  Constant/1 -> Out1/1
  Constant1/1 -> Out2/1

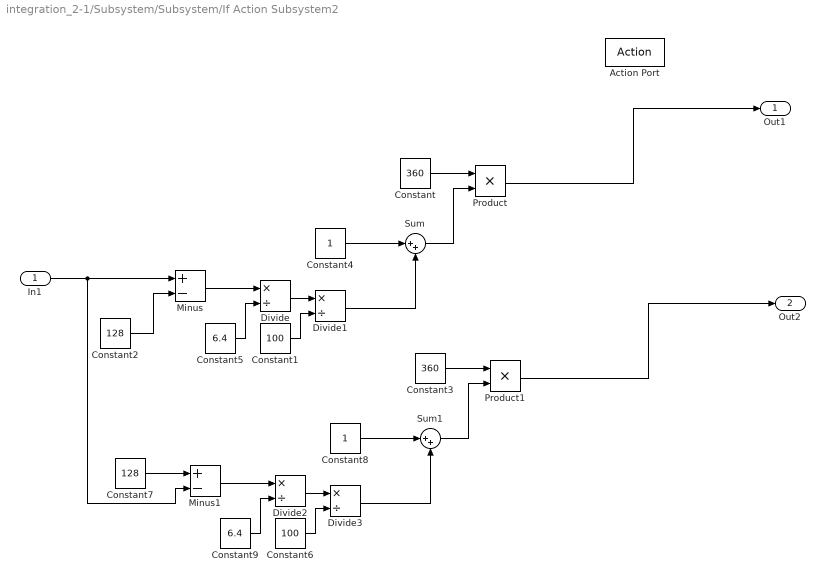
== system integration_2-1/Subsystem/Subsystem/If Action Subsystem2 ==
  In1 : Inport
  Action Port : ActionPort  ActionPortLabel=if(u1 ==0)
  Constant : Constant  Value=360
  Constant1 : Constant  Value=100
  Constant2 : Constant  Value=128
  Constant3 : Constant  Value=360
  Constant4 : Constant
  Constant5 : Constant  Value=6.4
  Constant6 : Constant  Value=100
  Constant7 : Constant  Value=128
  Constant8 : Constant
  Constant9 : Constant  Value=6.4
  Divide{,1..3} (4 alike) : Product  Inputs=*/
  Minus : Sum  Inputs=+-
  Minus1 : Sum  Inputs=+-
  Product : Product
  Product1 : Product
  Sum : Sum  Inputs=|++
  Sum1 : Sum  Inputs=|++
  Out1 : Outport
  Out2 : Outport  Port=2
  wires:
  Product/1 -> Out1/1
  Constant/1 -> Product/1
  In1/1 -> Minus/1, Minus1/2
  Constant2/1 -> Minus/2
  Minus/1 -> Divide/1
  Constant5/1 -> Divide/2
  Divide/1 -> Divide1/1
  Constant1/1 -> Divide1/2
  Constant4/1 -> Sum/1
  Divide1/1 -> Sum/2
  Sum/1 -> Product/2
  Constant7/1 -> Minus1/1
  Minus1/1 -> Divide2/1
  Constant3/1 -> Product1/1
  Constant9/1 -> Divide2/2
  Divide2/1 -> Divide3/1
  Divide3/1 -> Sum1/2
  Product1/1 -> Out2/1
  Constant6/1 -> Divide3/2
  Sum1/1 -> Product1/2
  Constant8/1 -> Sum1/1

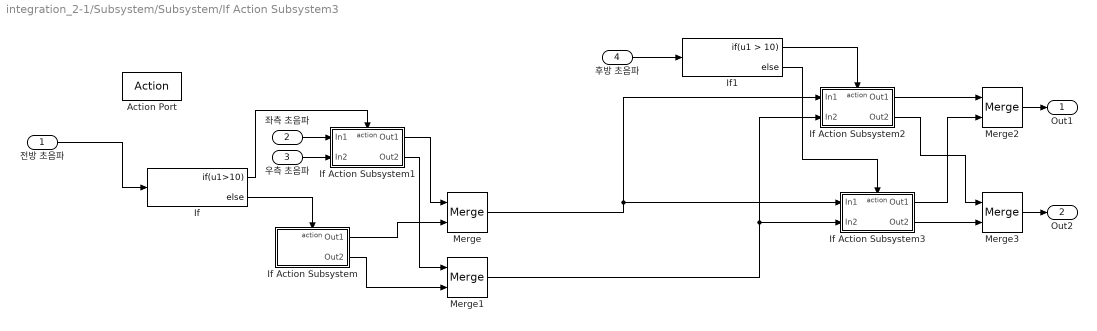
== system integration_2-1/Subsystem/Subsystem/If Action Subsystem3 ==
  전방 초음파 : Inport
  좌측 초음파 : Inport  Port=2
  우측 초음파 : Inport  Port=3
  후방 초음파 : Inport  Port=4
  Action Port : ActionPort  ActionPortLabel=else
  If : If  IfExpression=u1>10
  If Action Subsystem : Subsystem  TreatAsAtomicUnit=on
  If Action Subsystem1 : Subsystem  TreatAsAtomicUnit=on
  If Action Subsystem2 : Subsystem  TreatAsAtomicUnit=on
  If Action Subsystem3 : Subsystem  TreatAsAtomicUnit=on
  If1 : If  IfExpression=u1 > 10
  Merge{,1..3} (4 alike) : Merge
  Out1 : Outport
  Out2 : Outport  Port=2
  wires:
  If/2 -> If Action Subsystem/Action
  전방 초음파/1 -> If/1
  If/1 -> If Action Subsystem1/Action
  If Action Subsystem1/1(Out1) -> Merge/1
  If Action Subsystem/1(Out1) -> Merge/2
  Merge/1 -> If Action Subsystem3/1(In1), If Action Subsystem2/1(In1)
  If Action Subsystem1/2(Out2) -> Merge1/1
  If Action Subsystem/2(Out2) -> Merge1/2
  Merge1/1 -> If Action Subsystem3/2(In2), If Action Subsystem2/2(In2)
  좌측 초음파/1 -> If Action Subsystem1/1(In1)
  우측 초음파/1 -> If Action Subsystem1/2(In2)
  후방 초음파/1 -> If1/1
  If1/1 -> If Action Subsystem2/Action
  If1/2 -> If Action Subsystem3/Action
  If Action Subsystem2/1(Out1) -> Merge2/1
  If Action Subsystem3/1(Out1) -> Merge2/2
  If Action Subsystem3/2(Out2) -> Merge3/2
  If Action Subsystem2/2(Out2) -> Merge3/1
  Merge2/1 -> Out1/1
  Merge3/1 -> Out2/1

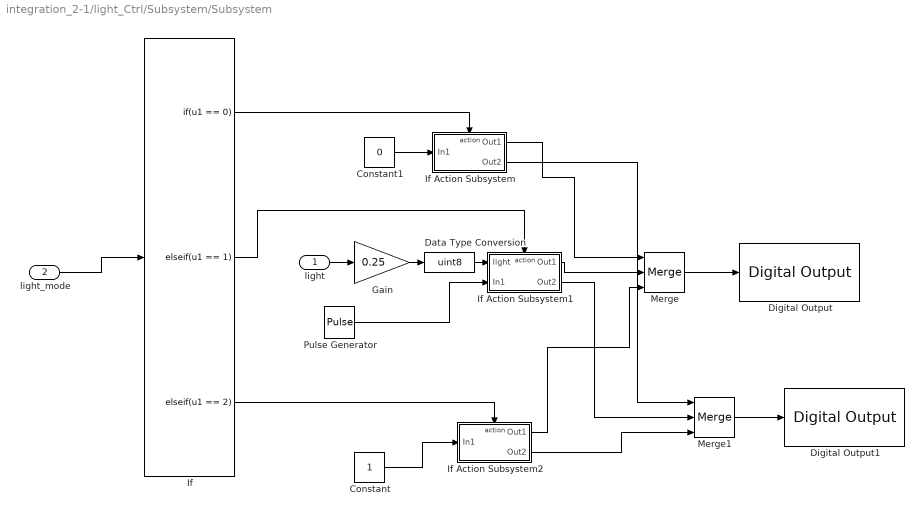
== system integration_2-1/light_Ctrl/Subsystem/Subsystem ==
  light : Inport
  light_mode : Inport  Port=2
  Constant : Constant
  Constant1 : Constant  Value=0
  Data Type Conversion : DataTypeConversion  OutDataTypeStr=uint8  SaturateOnIntegerOverflow=off  RndMeth=Floor
  Digital Output : arduinolib/Digital Output  pinNumber=LED2_R  Direction=output  blockPlatform=arduino
  Digital Output1 : arduinolib/Digital Output  pinNumber=LED2_B  Direction=output  blockPlatform=arduino
  Gain : Gain  Gain=0.25
  If : If  IfExpression=u1 == 0  ElseIfExpressions=u1 == 1, u1 == 2  ShowElse=off
  If Action Subsystem : Subsystem  TreatAsAtomicUnit=on
  If Action Subsystem1 : Subsystem  TreatAsAtomicUnit=on
  If Action Subsystem2 : Subsystem  TreatAsAtomicUnit=on
  Merge : Merge  Inputs=3
  Merge1 : Merge  Inputs=3
  Pulse Generator : DiscretePulseGenerator  PulseType=Time based  Period=0.2  PulseWidth=50
  wires:
  light_mode/1 -> If/1
  If/1 -> If Action Subsystem/Action
  If/2 -> If Action Subsystem1/Action
  If/3 -> If Action Subsystem2/Action
  Constant1/1 -> If Action Subsystem/1(In1)
  Constant/1 -> If Action Subsystem2/1(In1)
  If Action Subsystem/1(Out1) -> Merge/1
  If Action Subsystem1/1(Out1) -> Merge/2
  If Action Subsystem2/1(Out1) -> Merge/3
  Merge/1 -> Digital Output/1
  light/1 -> Gain/1
  Gain/1 -> Data Type Conversion/1
  Data Type Conversion/1 -> If Action Subsystem1/1(light)
  Pulse Generator/1 -> If Action Subsystem1/2(In1)
  If Action Subsystem1/2(Out2) -> Merge1/2
  If Action Subsystem/2(Out2) -> Merge1/1
  If Action Subsystem2/2(Out2) -> Merge1/3
  Merge1/1 -> Digital Output1/1

== system integration_2-1/Subsystem/Subsystem/If Action Subsystem3/If Action Subsystem ==
  Action Port : ActionPort  ActionPortLabel=else
  Constant : Constant  Value=0
  Constant1 : Constant  Value=0
  Out1 : Outport
  Out2 : Outport  Port=2
  wires:
  Constant1/1 -> Out2/1
  Constant/1 -> Out1/1

== system integration_2-1/Subsystem/Subsystem/If Action Subsystem3/If Action Subsystem1 ==
  In1 : Inport
  In2 : Inport  Port=2
  Action Port : ActionPort  ActionPortLabel=if(u1>10)
  If : If  NumInputs=2  IfExpression=(u1<10)&(u2<10)  ElseIfExpressions=u1<10,u2<10
  If Action Subsystem : Subsystem  TreatAsAtomicUnit=on
  If Action Subsystem1 : Subsystem  TreatAsAtomicUnit=on
  If Action Subsystem2 : Subsystem  TreatAsAtomicUnit=on
  If Action Subsystem3 : Subsystem  TreatAsAtomicUnit=on
  Merge : Merge  Inputs=4
  Merge1 : Merge  Inputs=4
  Out1 : Outport
  Out2 : Outport  Port=2
  wires:
  In1/1 -> If Action Subsystem1/1(In3), If Action Subsystem/1(In3), If/1
  If/1 -> If Action Subsystem/Action
  In2/1 -> If Action Subsystem2/1(In3), If Action Subsystem/2(In4), If/2
  If/2 -> If Action Subsystem1/Action
  If/3 -> If Action Subsystem2/Action
  If/4 -> If Action Subsystem3/Action
  If Action Subsystem/1(Out1) -> Merge/1
  If Action Subsystem1/1(Out2) -> Merge/2
  If Action Subsystem2/1(Out2) -> Merge/3
  If Action Subsystem3/1(Out1) -> Merge/4
  If Action Subsystem/2(Out2) -> Merge1/1
  If Action Subsystem1/2(Out3) -> Merge1/2
  If Action Subsystem2/2(Out3) -> Merge1/3
  If Action Subsystem3/2(Out2) -> Merge1/4
  Merge/1 -> Out1/1
  Merge1/1 -> Out2/1

== system integration_2-1/Subsystem/Subsystem/If Action Subsystem3/If Action Subsystem2 ==
  In1 : Inport
  In2 : Inport  Port=2
  Action Port : ActionPort  ActionPortLabel=if(u1 > 10)
  Out1 : Outport
  Out2 : Outport  Port=2
  wires:
  In1/1 -> Out1/1
  In2/1 -> Out2/1

== system integration_2-1/Subsystem/Subsystem/If Action Subsystem3/If Action Subsystem3 ==
  In1 : Inport
  In2 : Inport  Port=2
  Action Port : ActionPort  ActionPortLabel=else
  Gain : Gain  Gain=1.2
  Gain1 : Gain  Gain=1.2
  Out1 : Outport
  Out2 : Outport  Port=2
  wires:
  In1/1 -> Gain/1
  Gain/1 -> Out1/1
  In2/1 -> Gain1/1
  Gain1/1 -> Out2/1

== system integration_2-1/light_Ctrl/Subsystem/Subsystem/If Action Subsystem ==
  In1 : Inport
  Action Port : ActionPort  ActionPortLabel=if(u1 == 0)
  Out1 : Outport
  Out2 : Outport  Port=2
  wires:
  In1/1 -> Out2/1, Out1/1

== system integration_2-1/light_Ctrl/Subsystem/Subsystem/If Action Subsystem1 ==
  light : Inport
  In1 : Inport  Port=2
  Action Port : ActionPort  ActionPortLabel=elseif(u1 == 1)
  Constant : Constant
  Constant1 : Constant  Value=0
  If : If  IfExpression=u1 <= 150
  If Action Subsystem : Subsystem  TreatAsAtomicUnit=on
  If Action Subsystem1 : Subsystem  TreatAsAtomicUnit=on
  Merge : Merge
  Out1 : Outport
  Out2 : Outport  Port=2
  wires:
  light/1 -> If/1
  Constant/1 -> If Action Subsystem/1(In1)
  Constant1/1 -> If Action Subsystem1/1(In1)
  If/1 -> If Action Subsystem/Action
  If/2 -> If Action Subsystem1/Action
  If Action Subsystem/1(Out1) -> Merge/1
  If Action Subsystem1/1(Out1) -> Merge/2
  Merge/1 -> Out1/1
  In1/1 -> Out2/1

== system integration_2-1/light_Ctrl/Subsystem/Subsystem/If Action Subsystem2 ==
  In1 : Inport
  Action Port : ActionPort  ActionPortLabel=elseif( u1 == 2)
  Out1 : Outport
  Out2 : Outport  Port=2
  wires:
  In1/1 -> Out2/1, Out1/1

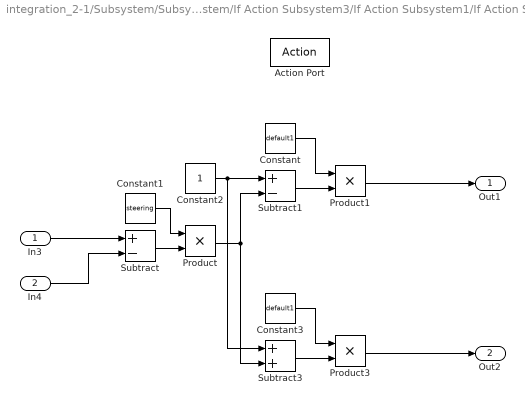
== system integration_2-1/Subsystem/Subsystem/If Action Subsystem3/If Action Subsystem1/If Action Subsystem ==
  In3 : Inport
  In4 : Inport  Port=2
  Action Port : ActionPort  ActionPortLabel=if((u1<10)&(u2<10))
  Constant : Constant  Value=default1
  Constant1 : Constant  Value=steering
  Constant2 : Constant
  Constant3 : Constant  Value=default1
  Product : Product
  Product1 : Product
  Product3 : Product
  Subtract : Sum  Inputs=+-
  Subtract1 : Sum  Inputs=+-
  Subtract3 : Sum
  Out1 : Outport
  Out2 : Outport  Port=2
  wires:
  Subtract/1 -> Product/2
  Constant1/1 -> Product/1
  Subtract1/1 -> Product1/2
  Product/1 -> Subtract1/2, Subtract3/2
  Constant/1 -> Product1/1
  Product1/1 -> Out1/1
  Subtract3/1 -> Product3/2
  Constant2/1 -> Subtract3/1, Subtract1/1
  In4/1 -> Subtract/2
  Constant3/1 -> Product3/1
  In3/1 -> Subtract/1
  Product3/1 -> Out2/1

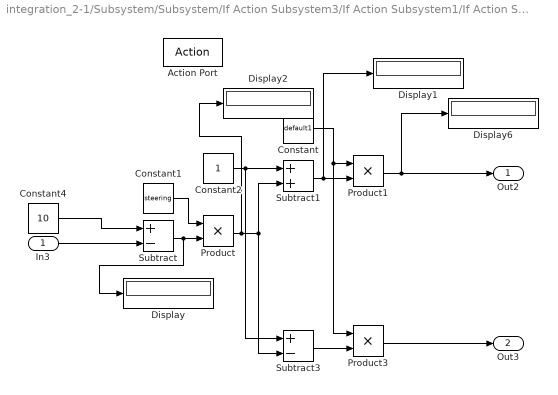
== system integration_2-1/Subsystem/Subsystem/If Action Subsystem3/If Action Subsystem1/If Action Subsystem1 ==
  In3 : Inport
  Action Port : ActionPort  ActionPortLabel=elseif(u1<10)
  Constant : Constant  Value=default1
  Constant1 : Constant  Value=steering
  Constant2 : Constant
  Constant4 : Constant  Value=10
  Display{,1..2,6} (4 alike) : Display
  Product : Product  OutDataTypeStr=double  RndMeth=Convergent
  Product1 : Product  OutDataTypeStr=double  RndMeth=Convergent
  Product3 : Product  OutDataTypeStr=double  RndMeth=Convergent
  Subtract : Sum  Inputs=+-  OutDataTypeStr=double  RndMeth=Convergent
  Subtract1 : Sum  OutDataTypeStr=double  RndMeth=Convergent
  Subtract3 : Sum  Inputs=+-  OutDataTypeStr=double  RndMeth=Convergent
  Out2 : Outport
  Out3 : Outport  Port=2
  wires:
  Product/1 -> Display2/1, Subtract1/2, Subtract3/2
  Subtract1/1 -> Display1/1, Product1/2
  Constant1/1 -> Product/1
  Constant2/1 -> Subtract3/1, Subtract1/1
  In3/1 -> Subtract/2
  Subtract/1 -> Display/1, Product/2
  Subtract3/1 -> Product3/2
  Product3/1 -> Out3/1
  Constant/1 -> Product3/1, Product1/1
  Product1/1 -> Display6/1, Out2/1
  Constant4/1 -> Subtract/1

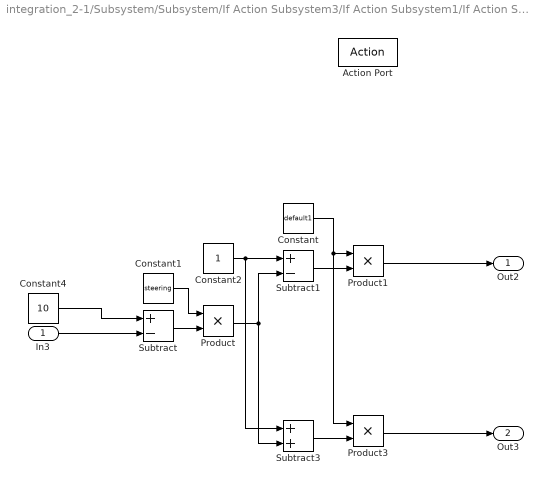
== system integration_2-1/Subsystem/Subsystem/If Action Subsystem3/If Action Subsystem1/If Action Subsystem2 ==
  In3 : Inport
  Action Port : ActionPort  ActionPortLabel=elseif(u2<10)
  Constant : Constant  Value=default1
  Constant1 : Constant  Value=steering
  Constant2 : Constant
  Constant4 : Constant  Value=10
  Product : Product
  Product1 : Product
  Product3 : Product
  Subtract : Sum  Inputs=+-
  Subtract1 : Sum  Inputs=+-
  Subtract3 : Sum
  Out2 : Outport
  Out3 : Outport  Port=2
  wires:
  Constant4/1 -> Subtract/1
  Constant/1 -> Product3/1, Product1/1
  Product/1 -> Subtract1/2, Subtract3/2
  Product3/1 -> Out3/1
  Subtract3/1 -> Product3/2
  Subtract/1 -> Product/2
  Subtract1/1 -> Product1/2
  Product1/1 -> Out2/1
  Constant1/1 -> Product/1
  Constant2/1 -> Subtract3/1, Subtract1/1
  In3/1 -> Subtract/2

== system integration_2-1/Subsystem/Subsystem/If Action Subsystem3/If Action Subsystem1/If Action Subsystem3 ==
  Action Port : ActionPort  ActionPortLabel=else
  Constant : Constant  Value=360
  Constant1 : Constant  Value=360
  Out1 : Outport
  Out2 : Outport  Port=2
  wires:
  Constant/1 -> Out1/1
  Constant1/1 -> Out2/1

== system integration_2-1/light_Ctrl/Subsystem/Subsystem/If Action Subsystem1/If Action Subsystem ==
  In1 : Inport
  Action Port : ActionPort  ActionPortLabel=if(u1 <= 150)
  Out1 : Outport
  wires:
  In1/1 -> Out1/1

== system integration_2-1/light_Ctrl/Subsystem/Subsystem/If Action Subsystem1/If Action Subsystem1 ==
  In1 : Inport
  Action Port : ActionPort  ActionPortLabel=else
  Out1 : Outport
  wires:
  In1/1 -> Out1/1

== stateflow chart integration_2-1/State_Ctrl/ADAS_state/If Action Subsystem/Chart ==
  state adas_off
    en,du:
    ADAS_state = sw2;
    state_2 = sw2;
  state adas_on
    en,du:
    ADAS_state = sw2;
    state_2 =sw2;
  (default) -> adas_off
  adas_off -> adas_on : [state_2 ~= sw2]
  adas_on -> adas_off : [state_2 ~= sw2]
  data: sw2 input; state_2 local; ADAS_state output

== stateflow chart integration_2-1/State_Ctrl/drive_mode/Chart ==
  state Drive_off
    en, du:
    drive_mode = 0;
    state_1 = sw1;
  state Drive_on
    en,du:
    drive_mode =1;
    state_1 = sw1;
    ADAS_state = A_state;
    Light_state = light_mode;
  (default) -> Drive_off
  Drive_off -> Drive_on : [state_1 ~= sw1]
  Drive_on -> Drive_off : [(state_1~=sw1) && (ADAS_state == 0) && (Light_state == 0)]
  data: sw1 input; light_mode input; state_1 local; drive_mode output; A_state input; ADAS_state local; Light_state local

== stateflow chart integration_2-1/light_Ctrl/Subsystem/Chart1 ==
  state light_auto
    en, du:
    light_mode = 1;
    state_1 = sw3;
  state light_off
    en, du:
    light_mode =0;
    state_1 = sw3;
  state light_on
    en,du:
    light_mode =2;
    state_1 = sw3;
  light_auto -> (junction 15) : [(state_1 ~= sw3) && (Drive_mode == 1)]
  (junction 12) -> light_auto
  (junction 15) -> light_on
  light_off -> (junction 12) : [(state_1 ~= sw3) && (Drive_mode == 1)]
  (default) -> light_off
  light_on -> light_off : [(state_1 ~= sw3) && (Drive_mode == 1)]
  data: sw3 input; Drive_mode input; state_1 local; light_mode output
